simulink model "simulink_example"  (R2019b)
settings: Solver=FixedStepAuto  StartTime=0.0  StopTime=inf  RelTol=1e-3
undefined symbols (not defined in the file or in its folder): f
libraries: instrumentlib x2, simulink x1
settings Model: Creator=Somers  LastModifiedBy=Somers

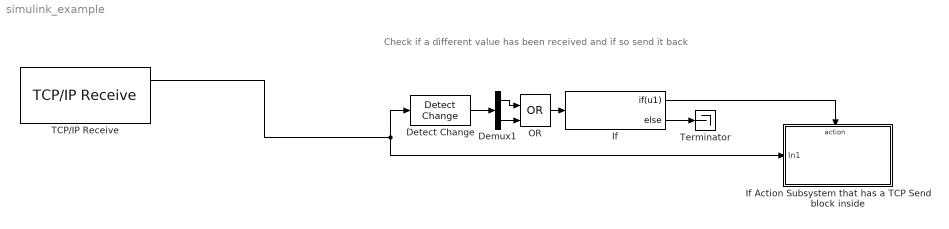
== system simulink_example ==
  note: Check if a different value has been received and if so send it back
  Demux1 : Demux  Outputs=2
  Detect Change : simulink/Logic and Bit Operations/Detect Change  vinit=0  OutDataTypeStr=uint8
  If : If  IfExpression=u1
  If Action Subsystem that has a TCP Send block inside : Subsystem  TreatAsAtomicUnit=on
  OR : Logic  Operator=OR  IconShape=distinctive  AllPortsSameDT=off  OutDataTypeStr=boolean
  TCP/IP Receive : instrumentlib/TCP//IP Receive  Host=127.0.0.1  Port=4242  DataSize=2  EnableBlockingMode=off  Timeout=10  SampleTime=0.01  DataType=single  ByteOrder=LittleEndian  ASCIIFormatting=%f,  Terminator=LF
      settings: SourceProductName=Instrument Control Toolbox
  Terminator : Terminator
  wires:
  If/2 -> Terminator/1
  TCP/IP Receive/1 -> Detect Change/1, If Action Subsystem that has a TCP Send block inside/1(In1)
  If/1 -> If Action Subsystem that has a TCP Send block inside/Action
  Detect Change/1 -> Demux1/1
  OR/1 -> If/1
  Demux1/1 -> OR/1
  Demux1/2 -> OR/2

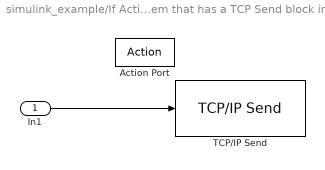
== system simulink_example/If Action Subsystem that has a TCP Send block inside ==
  In1 : Inport
  Action Port : ActionPort  ActionPortLabel=if(u1)
  TCP/IP Send : instrumentlib/TCP//IP Send  Host=127.0.0.1  Port=4343  EnableBlockingMode=off  Timeout=10  ByteOrder=LittleEndian  TransferDelay=off
      settings: SourceProductName=Instrument Control Toolbox
  wires:
  In1/1 -> TCP/IP Send/1
